simulink model "rigPeripheralNet"  (R2012b)
settings: Solver=FixedStepDiscrete  StartTime=0.0  StopTime=10.0  FixedStep=0.001  RelTol=1e-3
undefined symbols (not defined in the file): macaddr, modelConstants
libraries: xpcethernetlib x17, dspmtrx3 x6, simulink x5, xpcnetworkbufferlib x4, Lib_FileLogger x1
(part 1 of 2)
settings Model: xpc_rtwmakecfg_data=_xpcetherlib__xpcether8255xlib__xpcetherGbElib__xpcnblib_  BufferReuse=off  Creator=gilja  LastModifiedBy=NPTL
settings SolverCC: EnableConcurrentExecution=on  ConcurrentTasks=on
settings DataIOCC: SaveOutput=off  SignalLogging=off  SaveTime=off
settings OptimizationCC: InlineParams=on  InlineInvariantSignals=on  OptimizeBlockIOStorage=off  BufferReuse=off  ExpressionFolding=off  LocalBlockOutputs=off  SimCompilerOptimization=On
settings HardwareCC: ProdIntDivRoundTo=Zero  ProdEndianess=LittleEndian  ProdHWDeviceType=Generic->32-bit x86 compatible
settings ModelReferenceCC: ModelReferenceNumInstancesAllowed=Single  ModelReferenceMinAlgLoopOccurrences=on
settings RTWCC: SystemTargetFile=xpctarget.tlc  TemplateMakefile=xpc_default_tmf  Description=xPC Target  ProcessScript=xpctarget_make_rtw_hook  RTWCompilerOptimization=On
settings CodeAppCC: MaxIdLength=62
settings xpcTargetCC: TargetFcnLib=ansi_tfl_table_tmw.mat  CodeReplacementLibrary=XPC_BLAS  ParMdlRefBuildCompliant=on  ConcurrentExecutionCompliant=on  CombineSignalStateStructs=off  GRTInterface=on  xPCTaskExecutionProfile=on  xPCRL32EventNumber=5000  xPCisDownloadable=off  xPCLoadParamSetFile=off  xPCConcurrentTasks=off  xPCEnableSFAnimation=off

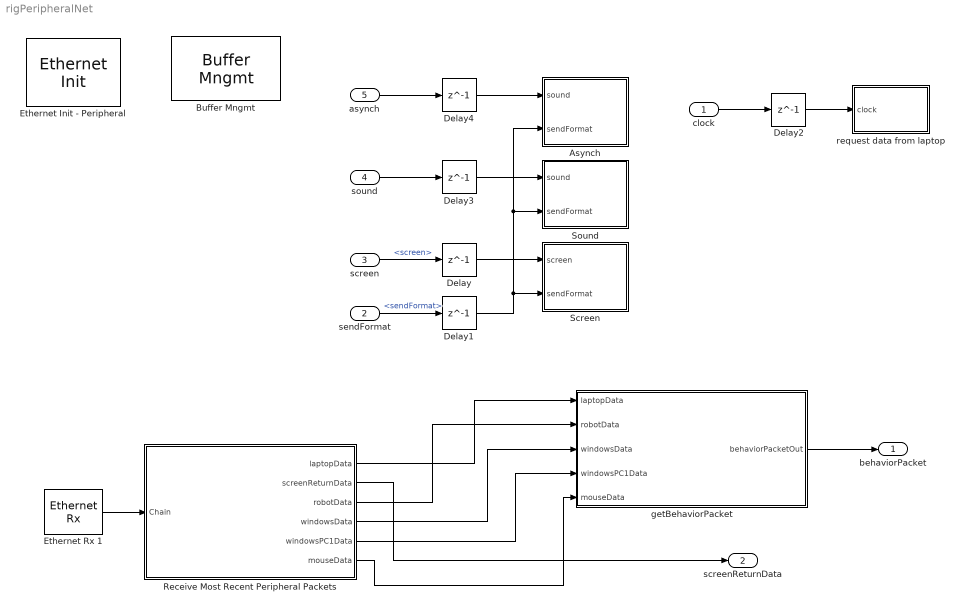
== system rigPeripheralNet ==
  clock : Inport  OutDataTypeStr=uint32
  sendFormat : Inport  Port=2  OutDataTypeStr=boolean
  screen : Inport  Port=3  OutDataTypeStr=Bus: fileLoggerFormatAndData  BusOutputAsStruct=on
  sound : Inport  Port=4  OutDataTypeStr=Bus: fileLoggerFormatAndData  BusOutputAsStruct=on
  asynch : Inport  Port=5  OutDataTypeStr=Bus: fileLoggerFormatAndData  BusOutputAsStruct=on
  Asynch : Subsystem
  "Buffer Mngmt " : xpcnetworkbufferlib/Buffer Mngmt   Priority=-1  SampleTime=-1  PoolSizes=modelConstants.networkBufferPoolSizes  ShowTune=on
  Delay{,1..4} (5 alike) : Delay  DelayLength=1  InitialCondition=0
  Ethernet Init - Peripheral : xpcethernetlib/Ethernet Init   Priority=-1  ID=3  Driver=Intel Gigabit  Bus=modelConstants.xpcNICConfig.peripheral.bus  Slot=modelConstants.xpcNICConfig.peripheral.slot  SampleTime=-1  AddressSource=Specify  MAC=macaddr('00:00:00:00:00:00')  TxSA=off  RxPromiscuous=off  Multicast={}  RxBad=off  RxShort=off  MaxMTU=1518  TxThreshold=10  TxBuffers=128  RxBuffers=8  ShowTune=on  NumRxBlks=1
  Ethernet Rx 1 : xpcethernetlib/Ethernet Rx   ID=3  SampleTime=modelConstants.sampleTime  Criteria=Receive all unmatched types [0 to 65535]  EtherType=[hex2dec('0000')]  BlkID=0
  Receive Most Recent Peripheral Packets : Subsystem
  Screen : Subsystem
  Sound : Subsystem
  getBehaviorPacket : MATLAB Function  TreatAsAtomicUnit=on
  request data from laptop : Subsystem
  behaviorPacket : Outport  OutDataTypeStr=Bus: behaviorPacketBus  BusOutputAsStruct=on
  screenReturnData : Outport  Port=2  OutDataTypeStr=Bus: peripheralData  BusOutputAsStruct=on
  wires:
  Ethernet Rx 1/1 -> Receive Most Recent Peripheral Packets/1(Chain)
  clock/1 -> Delay2/1
  Receive Most Recent Peripheral Packets/2(screenReturnData) -> screenReturnData/1
  sendFormat/1 -> Delay1/1  "<sendFormat>"
  screen/1 -> Delay/1  "<screen>"
  Delay/1 -> Screen/1(screen)
  Delay1/1 -> Asynch/2(sendFormat), Sound/2(sendFormat), Screen/2(sendFormat)
  Delay2/1 -> request data from laptop/1(clock)
  sound/1 -> Delay3/1
  Delay3/1 -> Sound/1(sound)
  asynch/1 -> Delay4/1
  Delay4/1 -> Asynch/1(sound)
  Receive Most Recent Peripheral Packets/1(laptopData) -> getBehaviorPacket/1(laptopData)
  Receive Most Recent Peripheral Packets/3(robotData) -> getBehaviorPacket/2(robotData)
  getBehaviorPacket/1(behaviorPacketOut) -> behaviorPacket/1
  Receive Most Recent Peripheral Packets/4(windowsData) -> getBehaviorPacket/3(windowsData)
  Receive Most Recent Peripheral Packets/5(windowsPC1Data) -> getBehaviorPacket/4(windowsPC1Data)
  Receive Most Recent Peripheral Packets/6(mouseData) -> getBehaviorPacket/5(mouseData)

== system rigPeripheralNet/Asynch ==
  sound : Inport  OutDataTypeStr=Bus: fileLoggerFormatAndData
  sendFormat : Inport  Port=2  OutDataTypeStr=boolean
  Asynch - Control : Subsystem
  Asynch - Data : Subsystem
  Bus Selector6 : BusSelector  OutputSignals=data.send,data.data,data.dataLen,format.format,format.formatLen
  Digital Clock : DigitalClock  SampleTime=0.001
  Logical Operator : Logic  AllPortsSameDT=off  OutDataTypeStr=boolean
  Logical Operator1 : Logic  AllPortsSameDT=off  OutDataTypeStr=boolean
  Wait 100 ms : simulink/Logic and Bit Operations/Compare To Constant  relop=>  const=0.4  OutDataTypeStr=boolean
  wires:
  Bus Selector6/3 -> Asynch - Data/2(dataLen)  "<dataLen>"
  Bus Selector6/2 -> Asynch - Data/1(data)  "<data>"
  Bus Selector6/1 -> Logical Operator1/2  "<send>"
  Bus Selector6/5 -> Asynch - Control/2(dataLen)  "<formatLen>"
  sound/1 -> Bus Selector6/1
  Bus Selector6/4 -> Asynch - Control/1(data)  "<format>"
  sendFormat/1 -> Logical Operator/2
  Wait 100 ms/1 -> Logical Operator/1, Logical Operator1/1
  Digital Clock/1 -> Wait 100 ms/1
  Logical Operator/1 -> Asynch - Control/Enable
  Logical Operator1/1 -> Asynch - Data/Enable

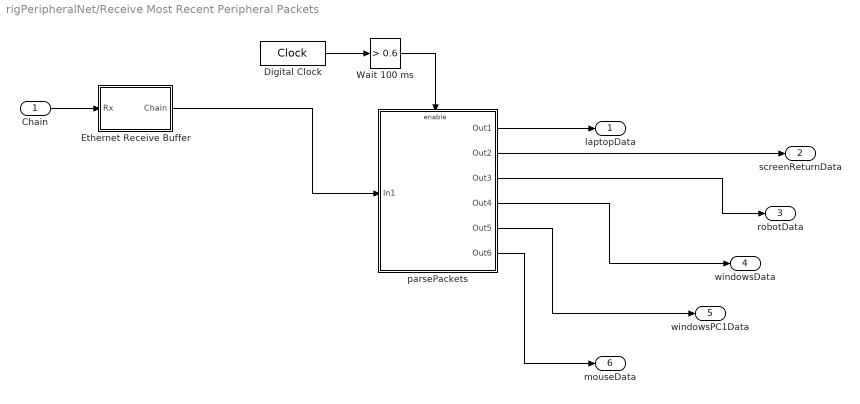
== system rigPeripheralNet/Receive Most Recent Peripheral Packets ==
  Chain : Inport
  Digital Clock : DigitalClock  SampleTime=0.001
  Ethernet Receive Buffer : Subsystem
  Wait 100 ms : simulink/Logic and Bit Operations/Compare To Constant  relop=>  const=0.6  OutDataTypeStr=boolean
  parsePackets : Subsystem
  laptopData : Outport  OutDataTypeStr=Bus: peripheralData
  screenReturnData : Outport  Port=2  OutDataTypeStr=Bus: peripheralData
  robotData : Outport  Port=3  OutDataTypeStr=Bus: peripheralData
  windowsData : Outport  Port=4  OutDataTypeStr=Bus: peripheralData
  windowsPC1Data : Outport  Port=5  OutDataTypeStr=Bus: peripheralData
  mouseData : Outport  Port=6  OutDataTypeStr=Bus: peripheralData
  wires:
  Chain/1 -> Ethernet Receive Buffer/1(Rx)
  Wait 100 ms/1 -> parsePackets/Enable
  Digital Clock/1 -> Wait 100 ms/1
  Ethernet Receive Buffer/1(Chain) -> parsePackets/1(In1)
  parsePackets/1(Out1) -> laptopData/1
  parsePackets/2(Out2) -> screenReturnData/1
  parsePackets/3(Out3) -> robotData/1
  parsePackets/4(Out4) -> windowsData/1
  parsePackets/5(Out5) -> windowsPC1Data/1
  parsePackets/6(Out6) -> mouseData/1

== system rigPeripheralNet/Screen ==
  screen : Inport  OutDataTypeStr=Bus: fileLoggerFormatAndData
  sendFormat : Inport  Port=2  OutDataTypeStr=boolean
  Bus Selector6 : BusSelector  OutputSignals=data.send,data.data,data.dataLen,format.format,format.formatLen
  Digital Clock : DigitalClock  SampleTime=0.001
  Logical Operator : Logic  AllPortsSameDT=off  OutDataTypeStr=boolean
  Logical Operator1 : Logic  AllPortsSameDT=off  OutDataTypeStr=boolean
  Screen - Control : Subsystem
  Screen - Data : Subsystem
  Wait 400 ms xPC has memory intialization issues early in the task : simulink/Logic and Bit Operations/Compare To Constant  relop=>  const=0.4  OutDataTypeStr=boolean
  wires:
  Bus Selector6/3 -> Screen - Data/2(dataLen)  "<dataLen>"
  Bus Selector6/2 -> Screen - Data/1(data)  "<data>"
  Bus Selector6/1 -> Logical Operator/2  "<send>"
  Bus Selector6/5 -> Screen - Control/2(dataLen)  "<formatLen>"
  screen/1 -> Bus Selector6/1
  Bus Selector6/4 -> Screen - Control/1(data)  "<format>"
  sendFormat/1 -> Logical Operator1/2
  Logical Operator/1 -> Screen - Data/Enable
  Logical Operator1/1 -> Screen - Control/Enable
  Digital Clock/1 -> Wait 400 ms xPC has memory intialization issues early in the task/1
  Wait 400 ms xPC has memory intialization issues early in the task/1 -> Logical Operator1/1, Logical Operator/1

== system rigPeripheralNet/Sound ==
  sound : Inport  OutDataTypeStr=Bus: fileLoggerFormatAndData
  sendFormat : Inport  Port=2  OutDataTypeStr=boolean
  Bus Selector6 : BusSelector  OutputSignals=data.send,data.data,data.dataLen,format.format,format.formatLen
  Digital Clock : DigitalClock  SampleTime=0.001
  Logical Operator : Logic  AllPortsSameDT=off  OutDataTypeStr=boolean
  Logical Operator1 : Logic  AllPortsSameDT=off  OutDataTypeStr=boolean
  Sound - Control : Subsystem
  Sound - Data : Subsystem
  Wait 100 ms : simulink/Logic and Bit Operations/Compare To Constant  relop=>  const=0.4  OutDataTypeStr=boolean
  wires:
  Bus Selector6/3 -> Sound - Data/2(dataLen)  "<dataLen>"
  Bus Selector6/2 -> Sound - Data/1(data)  "<data>"
  Bus Selector6/1 -> Logical Operator/2  "<send>"
  Bus Selector6/5 -> Sound - Control/2(dataLen)  "<formatLen>"
  sound/1 -> Bus Selector6/1
  Bus Selector6/4 -> Sound - Control/1(data)  "<format>"
  sendFormat/1 -> Logical Operator1/2
  Digital Clock/1 -> Wait 100 ms/1
  Wait 100 ms/1 -> Logical Operator1/1, Logical Operator/1
  Logical Operator/1 -> Sound - Data/Enable
  Logical Operator1/1 -> Sound - Control/Enable

== system rigPeripheralNet/request data from laptop ==
  clock : Inport
  Digital Clock : DigitalClock  SampleTime=0.001
  Laptop Data Request : MATLAB Function  TreatAsAtomicUnit=on
  Logical Operator : Logic  AllPortsSameDT=off  OutDataTypeStr=boolean
  UDP to Laptop : Subsystem
  Wait 100 ms : simulink/Logic and Bit Operations/Compare To Constant  relop=>  const=0.4  OutDataTypeStr=boolean
  wires:
  Laptop Data Request/3(dataLen) -> UDP to Laptop/2(udpDataLen)
  Laptop Data Request/2(data) -> UDP to Laptop/1(udpData)
  Logical Operator/1 -> UDP to Laptop/Enable
  clock/1 -> Laptop Data Request/1(clock)
  Digital Clock/1 -> Wait 100 ms/1
  Wait 100 ms/1 -> Logical Operator/1
  Laptop Data Request/1(send) -> Logical Operator/2

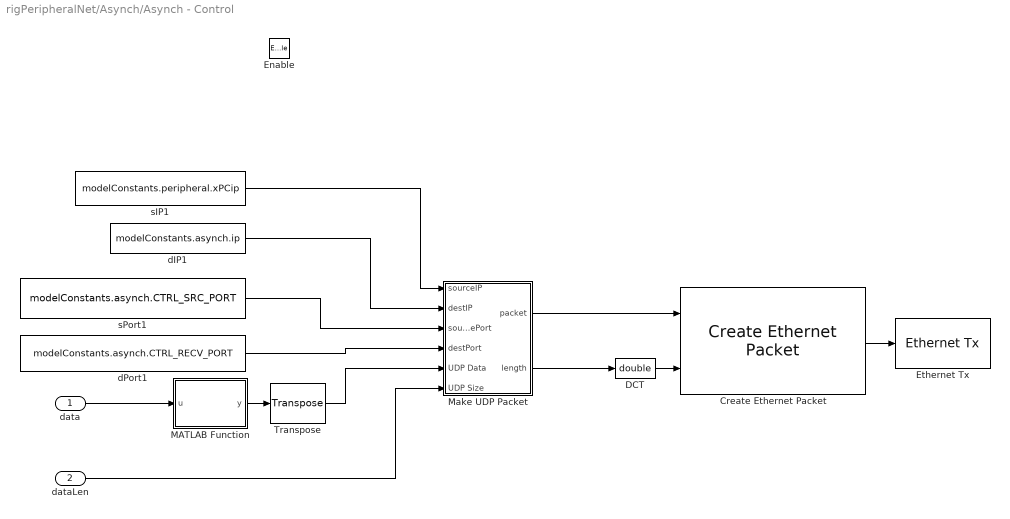
== system rigPeripheralNet/Asynch/Asynch - Control ==
  data : Inport
  dataLen : Inport  Port=2
  Enable : EnablePort
  "Create Ethernet Packet " : xpcethernetlib/Create Ethernet Packet   DstMac=macaddr('FF:FF:FF:FF:FF:FF')  EtherType=hex2dec('0800')
  DCT : DataTypeConversion  OutDataTypeStr=double
  "Ethernet Tx " : xpcethernetlib/Ethernet Tx   ID=3  SampleTime=-1
  MATLAB Function : MATLAB Function  TreatAsAtomicUnit=on
  Make UDP Packet : Subsystem
  Transpose : dspmtrx3/Transpose  Hermitian=off  overflowFlag=off
  dIP1 : Constant  Value=modelConstants.asynch.ip  OutDataTypeStr=uint8
  dPort1 : Constant  Value=modelConstants.asynch.CTRL_RECV_PORT  OutDataTypeStr=uint16
  sIP1 : Constant  Value=modelConstants.peripheral.xPCip  OutDataTypeStr=uint8
  sPort1 : Constant  Value=modelConstants.asynch.CTRL_SRC_PORT  OutDataTypeStr=uint16
  wires:
  dPort1/1 -> Make UDP Packet/4(destPort)
  Make UDP Packet/2(length) -> DCT/1
  "Create Ethernet Packet "/1 -> "Ethernet Tx "/1
  Make UDP Packet/1(packet) -> "Create Ethernet Packet "/1
  DCT/1 -> "Create Ethernet Packet "/2
  data/1 -> MATLAB Function/1(u)
  MATLAB Function/1(y) -> Transpose/1
  dataLen/1 -> Make UDP Packet/6(UDP Size)
  sPort1/1 -> Make UDP Packet/3(sourcePort)
  dIP1/1 -> Make UDP Packet/2(destIP)
  sIP1/1 -> Make UDP Packet/1(sourceIP)
  Transpose/1 -> Make UDP Packet/5(UDP Data)

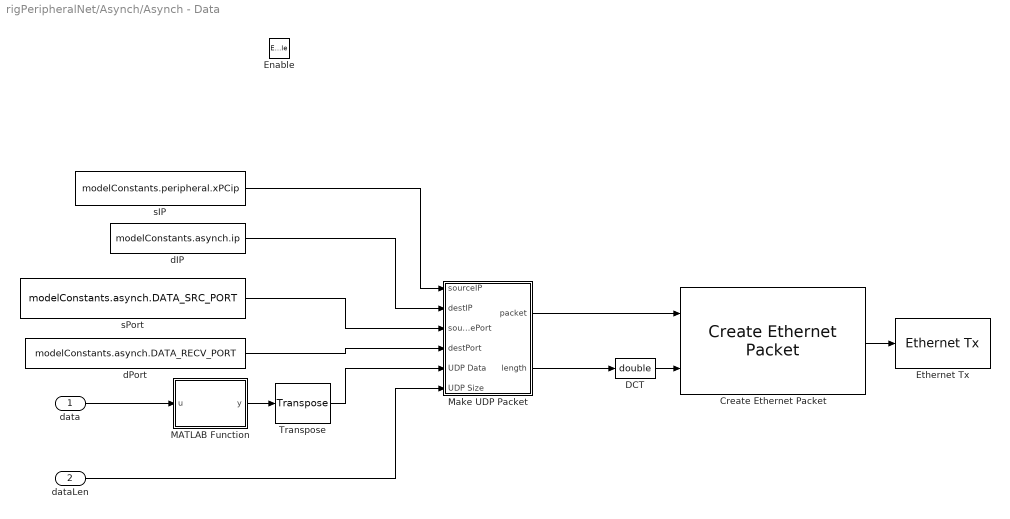
== system rigPeripheralNet/Asynch/Asynch - Data ==
  data : Inport
  dataLen : Inport  Port=2
  Enable : EnablePort
  "Create Ethernet Packet " : xpcethernetlib/Create Ethernet Packet   DstMac=macaddr('FF:FF:FF:FF:FF:FF')  EtherType=hex2dec('0800')
  DCT : DataTypeConversion  OutDataTypeStr=double
  "Ethernet Tx " : xpcethernetlib/Ethernet Tx   ID=3  SampleTime=-1
  MATLAB Function : MATLAB Function  TreatAsAtomicUnit=on
  Make UDP Packet : Subsystem
  Transpose : dspmtrx3/Transpose  Hermitian=off  overflowFlag=off
  dIP : Constant  Value=modelConstants.asynch.ip  OutDataTypeStr=uint8
  dPort : Constant  Value=modelConstants.asynch.DATA_RECV_PORT  OutDataTypeStr=uint16
  sIP : Constant  Value=modelConstants.peripheral.xPCip  OutDataTypeStr=uint8
  sPort : Constant  Value=modelConstants.asynch.DATA_SRC_PORT  OutDataTypeStr=uint16
  wires:
  dPort/1 -> Make UDP Packet/4(destPort)
  Make UDP Packet/2(length) -> DCT/1
  "Create Ethernet Packet "/1 -> "Ethernet Tx "/1
  Make UDP Packet/1(packet) -> "Create Ethernet Packet "/1
  DCT/1 -> "Create Ethernet Packet "/2
  data/1 -> MATLAB Function/1(u)
  MATLAB Function/1(y) -> Transpose/1
  dataLen/1 -> Make UDP Packet/6(UDP Size)
  sPort/1 -> Make UDP Packet/3(sourcePort)
  dIP/1 -> Make UDP Packet/2(destIP)
  sIP/1 -> Make UDP Packet/1(sourceIP)
  Transpose/1 -> Make UDP Packet/5(UDP Data)

== system rigPeripheralNet/Receive Most Recent Peripheral Packets/Ethernet Receive Buffer ==
  note: HACK: HARDCODED CHAIN BUFFER AT 39
      | Affects NB Buffering Block & NB Unlink
  Rx : Inport
  Buffer : xpcnetworkbufferlib/Buffer   ChainSize=38  BufferSize=0  Threshold=0
  Bus Creator : BusCreator  Inputs=2
  "Chain Size " : xpcnetworkbufferlib/Chain Size 
  Chain : Outport
  wires:
  Buffer/1 -> Bus Creator/1  "Buffers"
  Bus Creator/1 -> Chain/1
  "Chain Size "/2 -> Bus Creator/2  "Chain Size"
  Rx/1 -> "Chain Size "/1
  "Chain Size "/1 -> Buffer/1

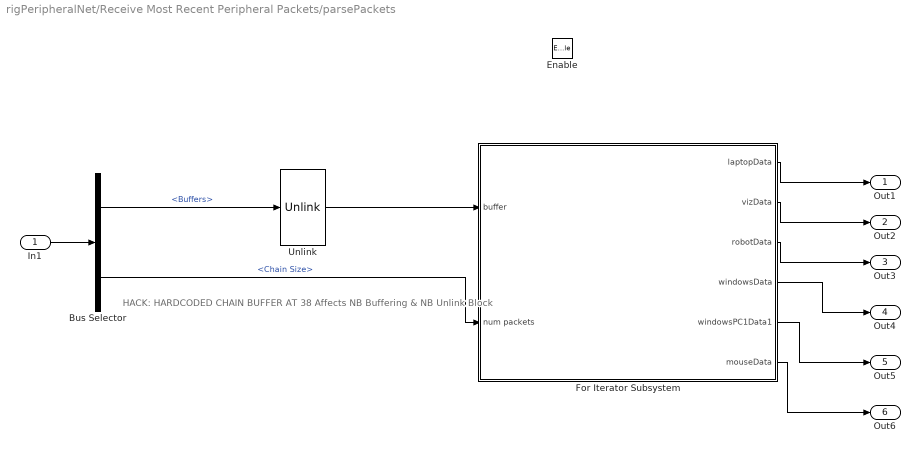
== system rigPeripheralNet/Receive Most Recent Peripheral Packets/parsePackets ==
  note: HACK: HARDCODED CHAIN BUFFER AT 38
      | Affects NB Buffering & NB Unlink Block
  In1 : Inport
  Enable : EnablePort
  Bus Selector : BusSelector  OutputSignals=Buffers,Chain Size
  For Iterator Subsystem : Subsystem  TreatAsAtomicUnit=on
  "Unlink " : xpcnetworkbufferlib/Unlink   VectorLength=38
  Out1 : Outport
  Out2 : Outport  Port=2
  Out3 : Outport  Port=3
  Out4 : Outport  Port=4
  Out5 : Outport  Port=5  OutDataTypeStr=Bus: peripheralData
  Out6 : Outport  Port=6  OutDataTypeStr=Bus: peripheralData
  wires:
  In1/1 -> Bus Selector/1
  For Iterator Subsystem/1(laptopData) -> Out1/1
  For Iterator Subsystem/2(vizData) -> Out2/1
  "Unlink "/1 -> For Iterator Subsystem/1(buffer)
  Bus Selector/1 -> "Unlink "/1  "<Buffers>"
  For Iterator Subsystem/3(robotData) -> Out3/1
  Bus Selector/2 -> For Iterator Subsystem/2(num packets)  "<Chain Size>"
  For Iterator Subsystem/4(windowsData) -> Out4/1
  For Iterator Subsystem/5(windowsPC1Data1) -> Out5/1
  For Iterator Subsystem/6(mouseData) -> Out6/1

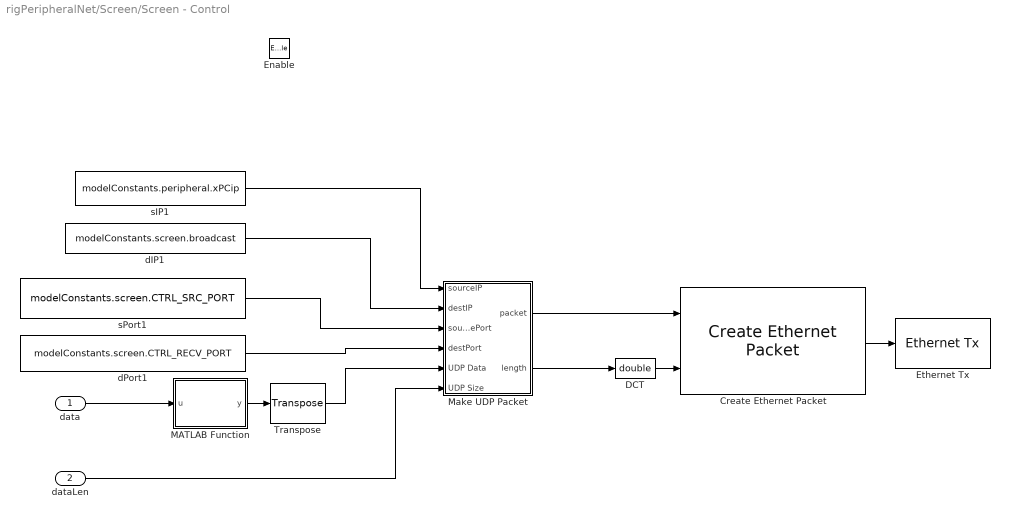
== system rigPeripheralNet/Screen/Screen - Control ==
  data : Inport
  dataLen : Inport  Port=2
  Enable : EnablePort
  "Create Ethernet Packet " : xpcethernetlib/Create Ethernet Packet   DstMac=macaddr('FF:FF:FF:FF:FF:FF')  EtherType=hex2dec('0800')
  DCT : DataTypeConversion  OutDataTypeStr=double
  "Ethernet Tx " : xpcethernetlib/Ethernet Tx   ID=3  SampleTime=-1
  MATLAB Function : MATLAB Function  TreatAsAtomicUnit=on
  Make UDP Packet : Subsystem
  Transpose : dspmtrx3/Transpose  Hermitian=off  overflowFlag=off
  dIP1 : Constant  Value=modelConstants.screen.broadcast  OutDataTypeStr=uint8
  dPort1 : Constant  Value=modelConstants.screen.CTRL_RECV_PORT  OutDataTypeStr=uint16
  sIP1 : Constant  Value=modelConstants.peripheral.xPCip  OutDataTypeStr=uint8
  sPort1 : Constant  Value=modelConstants.screen.CTRL_SRC_PORT  OutDataTypeStr=uint16
  wires:
  dPort1/1 -> Make UDP Packet/4(destPort)
  Make UDP Packet/2(length) -> DCT/1
  "Create Ethernet Packet "/1 -> "Ethernet Tx "/1
  Make UDP Packet/1(packet) -> "Create Ethernet Packet "/1
  DCT/1 -> "Create Ethernet Packet "/2
  data/1 -> MATLAB Function/1(u)
  MATLAB Function/1(y) -> Transpose/1
  dataLen/1 -> Make UDP Packet/6(UDP Size)
  sPort1/1 -> Make UDP Packet/3(sourcePort)
  dIP1/1 -> Make UDP Packet/2(destIP)
  sIP1/1 -> Make UDP Packet/1(sourceIP)
  Transpose/1 -> Make UDP Packet/5(UDP Data)

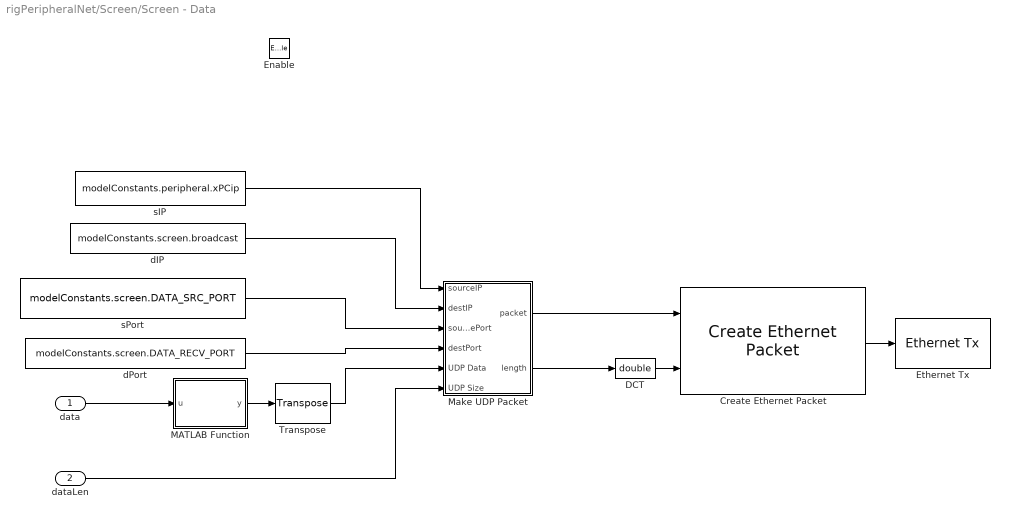
== system rigPeripheralNet/Screen/Screen - Data ==
  data : Inport
  dataLen : Inport  Port=2
  Enable : EnablePort
  "Create Ethernet Packet " : xpcethernetlib/Create Ethernet Packet   DstMac=macaddr('FF:FF:FF:FF:FF:FF')  EtherType=hex2dec('0800')
  DCT : DataTypeConversion  OutDataTypeStr=double
  "Ethernet Tx " : xpcethernetlib/Ethernet Tx   ID=3  SampleTime=-1
  MATLAB Function : MATLAB Function  TreatAsAtomicUnit=on
  Make UDP Packet : Subsystem
  Transpose : dspmtrx3/Transpose  Hermitian=off  overflowFlag=off
  dIP : Constant  Value=modelConstants.screen.broadcast  OutDataTypeStr=uint8
  dPort : Constant  Value=modelConstants.screen.DATA_RECV_PORT  OutDataTypeStr=uint16
  sIP : Constant  Value=modelConstants.peripheral.xPCip  OutDataTypeStr=uint8
  sPort : Constant  Value=modelConstants.screen.DATA_SRC_PORT  OutDataTypeStr=uint16
  wires:
  dPort/1 -> Make UDP Packet/4(destPort)
  Make UDP Packet/2(length) -> DCT/1
  "Create Ethernet Packet "/1 -> "Ethernet Tx "/1
  Make UDP Packet/1(packet) -> "Create Ethernet Packet "/1
  DCT/1 -> "Create Ethernet Packet "/2
  data/1 -> MATLAB Function/1(u)
  MATLAB Function/1(y) -> Transpose/1
  dataLen/1 -> Make UDP Packet/6(UDP Size)
  sPort/1 -> Make UDP Packet/3(sourcePort)
  dIP/1 -> Make UDP Packet/2(destIP)
  sIP/1 -> Make UDP Packet/1(sourceIP)
  Transpose/1 -> Make UDP Packet/5(UDP Data)

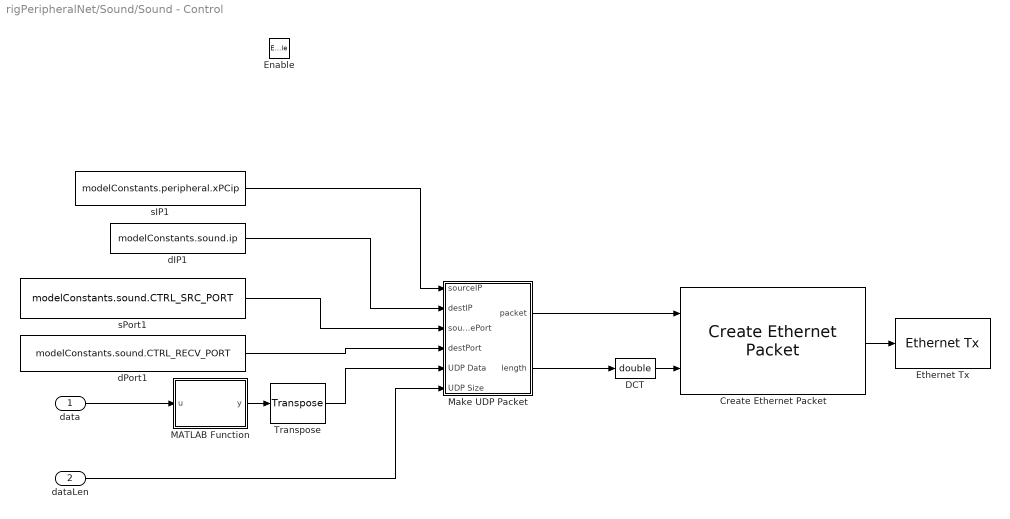
== system rigPeripheralNet/Sound/Sound - Control ==
  data : Inport
  dataLen : Inport  Port=2
  Enable : EnablePort
  "Create Ethernet Packet " : xpcethernetlib/Create Ethernet Packet   DstMac=macaddr('FF:FF:FF:FF:FF:FF')  EtherType=hex2dec('0800')
  DCT : DataTypeConversion  OutDataTypeStr=double
  "Ethernet Tx " : xpcethernetlib/Ethernet Tx   ID=3  SampleTime=-1
  MATLAB Function : MATLAB Function  TreatAsAtomicUnit=on
  Make UDP Packet : Subsystem
  Transpose : dspmtrx3/Transpose  Hermitian=off  overflowFlag=off
  dIP1 : Constant  Value=modelConstants.sound.ip  OutDataTypeStr=uint8
  dPort1 : Constant  Value=modelConstants.sound.CTRL_RECV_PORT  OutDataTypeStr=uint16
  sIP1 : Constant  Value=modelConstants.peripheral.xPCip  OutDataTypeStr=uint8
  sPort1 : Constant  Value=modelConstants.sound.CTRL_SRC_PORT  OutDataTypeStr=uint16
  wires:
  dPort1/1 -> Make UDP Packet/4(destPort)
  Make UDP Packet/2(length) -> DCT/1
  "Create Ethernet Packet "/1 -> "Ethernet Tx "/1
  Make UDP Packet/1(packet) -> "Create Ethernet Packet "/1
  DCT/1 -> "Create Ethernet Packet "/2
  data/1 -> MATLAB Function/1(u)
  MATLAB Function/1(y) -> Transpose/1
  dataLen/1 -> Make UDP Packet/6(UDP Size)
  sPort1/1 -> Make UDP Packet/3(sourcePort)
  dIP1/1 -> Make UDP Packet/2(destIP)
  sIP1/1 -> Make UDP Packet/1(sourceIP)
  Transpose/1 -> Make UDP Packet/5(UDP Data)

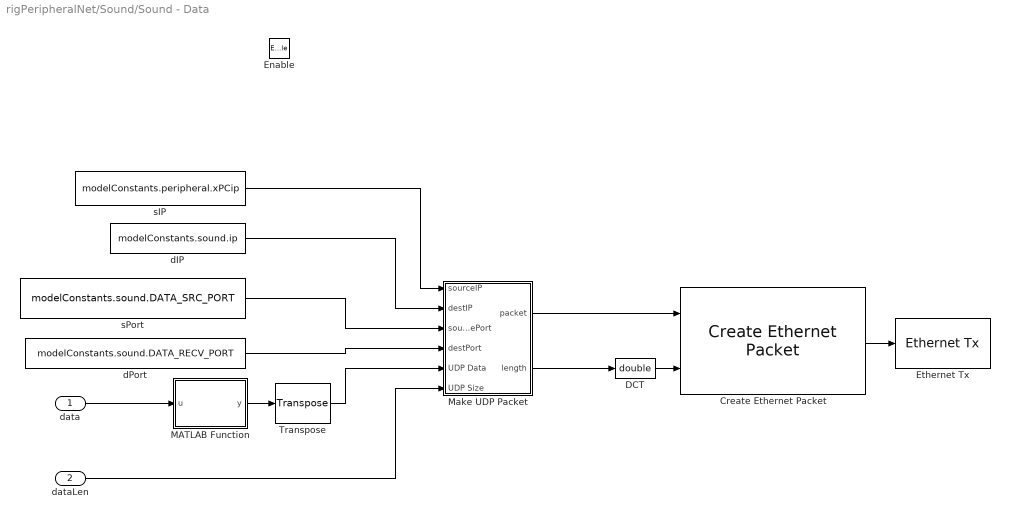
== system rigPeripheralNet/Sound/Sound - Data ==
  data : Inport
  dataLen : Inport  Port=2
  Enable : EnablePort
  "Create Ethernet Packet " : xpcethernetlib/Create Ethernet Packet   DstMac=macaddr('FF:FF:FF:FF:FF:FF')  EtherType=hex2dec('0800')
  DCT : DataTypeConversion  OutDataTypeStr=double
  "Ethernet Tx " : xpcethernetlib/Ethernet Tx   ID=3  SampleTime=-1
  MATLAB Function : MATLAB Function  TreatAsAtomicUnit=on
  Make UDP Packet : Subsystem
  Transpose : dspmtrx3/Transpose  Hermitian=off  overflowFlag=off
  dIP : Constant  Value=modelConstants.sound.ip  OutDataTypeStr=uint8
  dPort : Constant  Value=modelConstants.sound.DATA_RECV_PORT  OutDataTypeStr=uint16
  sIP : Constant  Value=modelConstants.peripheral.xPCip  OutDataTypeStr=uint8
  sPort : Constant  Value=modelConstants.sound.DATA_SRC_PORT  OutDataTypeStr=uint16
  wires:
  dPort/1 -> Make UDP Packet/4(destPort)
  Make UDP Packet/2(length) -> DCT/1
  "Create Ethernet Packet "/1 -> "Ethernet Tx "/1
  Make UDP Packet/1(packet) -> "Create Ethernet Packet "/1
  DCT/1 -> "Create Ethernet Packet "/2
  data/1 -> MATLAB Function/1(u)
  MATLAB Function/1(y) -> Transpose/1
  dataLen/1 -> Make UDP Packet/6(UDP Size)
  sPort/1 -> Make UDP Packet/3(sourcePort)
  dIP/1 -> Make UDP Packet/2(destIP)
  sIP/1 -> Make UDP Packet/1(sourceIP)
  Transpose/1 -> Make UDP Packet/5(UDP Data)

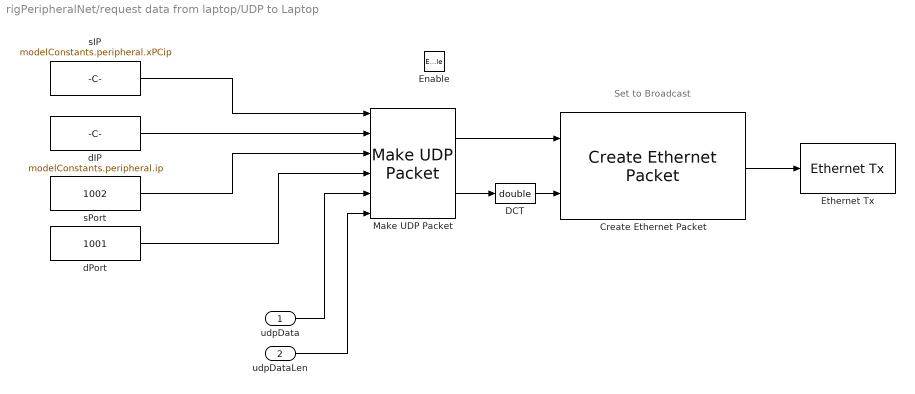
== system rigPeripheralNet/request data from laptop/UDP to Laptop ==
  note: Set to Broadcast
  udpData : Inport
  udpDataLen : Inport  Port=2
  Enable : EnablePort
  "Create Ethernet Packet " : xpcethernetlib/Create Ethernet Packet   DstMac=macaddr('FF:FF:FF:FF:FF:FF')  EtherType=hex2dec('0800')
  DCT : DataTypeConversion  OutDataTypeStr=double
  "Ethernet Tx " : xpcethernetlib/Ethernet Tx   ID=3  SampleTime=-1
  Make UDP Packet : Lib_FileLogger/Fille Logger/Make UDP Packet
  dIP : Constant  Value=modelConstants.peripheral.ip  OutDataTypeStr=uint8
  dPort : Constant  Value=1001  OutDataTypeStr=uint16
  sIP : Constant  Value=modelConstants.peripheral.xPCip  OutDataTypeStr=uint8
  sPort : Constant  Value=1002  OutDataTypeStr=uint16
  wires:
  dPort/1 -> Make UDP Packet/4
  sIP/1 -> Make UDP Packet/1
  Make UDP Packet/2 -> DCT/1
  Make UDP Packet/1 -> "Create Ethernet Packet "/1
  DCT/1 -> "Create Ethernet Packet "/2
  dIP/1 -> Make UDP Packet/2
  sPort/1 -> Make UDP Packet/3
  udpDataLen/1 -> Make UDP Packet/6
  "Create Ethernet Packet "/1 -> "Ethernet Tx "/1
  udpData/1 -> Make UDP Packet/5

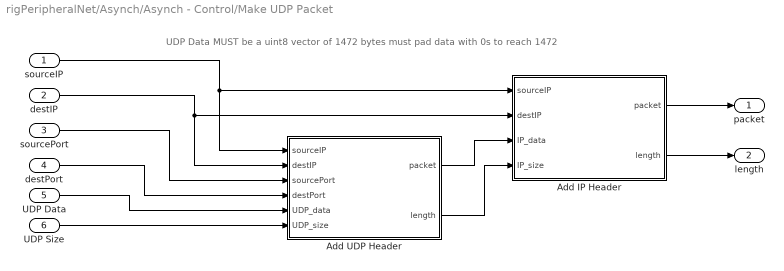
== system rigPeripheralNet/Asynch/Asynch - Control/Make UDP Packet ==
  note: UDP Data MUST be a uint8 vector of 1472 bytes
      | must pad data with 0s to reach 1472
  sourceIP : Inport
  destIP : Inport  Port=2
  sourcePort : Inport  Port=3
  destPort : Inport  Port=4
  UDP Data : Inport  Port=5
  UDP Size : Inport  Port=6
  Add IP Header : MATLAB Function  TreatAsAtomicUnit=on
  Add UDP Header : MATLAB Function  TreatAsAtomicUnit=on
  packet : Outport
  length : Outport  Port=2
  wires:
  Add UDP Header/2(length) -> Add IP Header/4(IP_size)
  Add UDP Header/1(packet) -> Add IP Header/3(IP_data)
  sourceIP/1 -> Add UDP Header/1(sourceIP), Add IP Header/1(sourceIP)
  destIP/1 -> Add UDP Header/2(destIP), Add IP Header/2(destIP)
  sourcePort/1 -> Add UDP Header/3(sourcePort)
  destPort/1 -> Add UDP Header/4(destPort)
  UDP Data/1 -> Add UDP Header/5(UDP_data)
  Add IP Header/1(packet) -> packet/1
  Add IP Header/2(length) -> length/1
  UDP Size/1 -> Add UDP Header/6(UDP_size)

== system rigPeripheralNet/Asynch/Asynch - Data/Make UDP Packet ==
  note: UDP Data MUST be a uint8 vector of 1472 bytes
      | must pad data with 0s to reach 1472
  sourceIP : Inport
  destIP : Inport  Port=2
  sourcePort : Inport  Port=3
  destPort : Inport  Port=4
  UDP Data : Inport  Port=5
  UDP Size : Inport  Port=6
  Add IP Header : MATLAB Function  TreatAsAtomicUnit=on
  Add UDP Header : MATLAB Function  TreatAsAtomicUnit=on
  packet : Outport
  length : Outport  Port=2
  wires:
  Add UDP Header/2(length) -> Add IP Header/4(IP_size)
  Add UDP Header/1(packet) -> Add IP Header/3(IP_data)
  sourceIP/1 -> Add UDP Header/1(sourceIP), Add IP Header/1(sourceIP)
  destIP/1 -> Add UDP Header/2(destIP), Add IP Header/2(destIP)
  sourcePort/1 -> Add UDP Header/3(sourcePort)
  destPort/1 -> Add UDP Header/4(destPort)
  UDP Data/1 -> Add UDP Header/5(UDP_data)
  Add IP Header/1(packet) -> packet/1
  Add IP Header/2(length) -> length/1
  UDP Size/1 -> Add UDP Header/6(UDP_size)

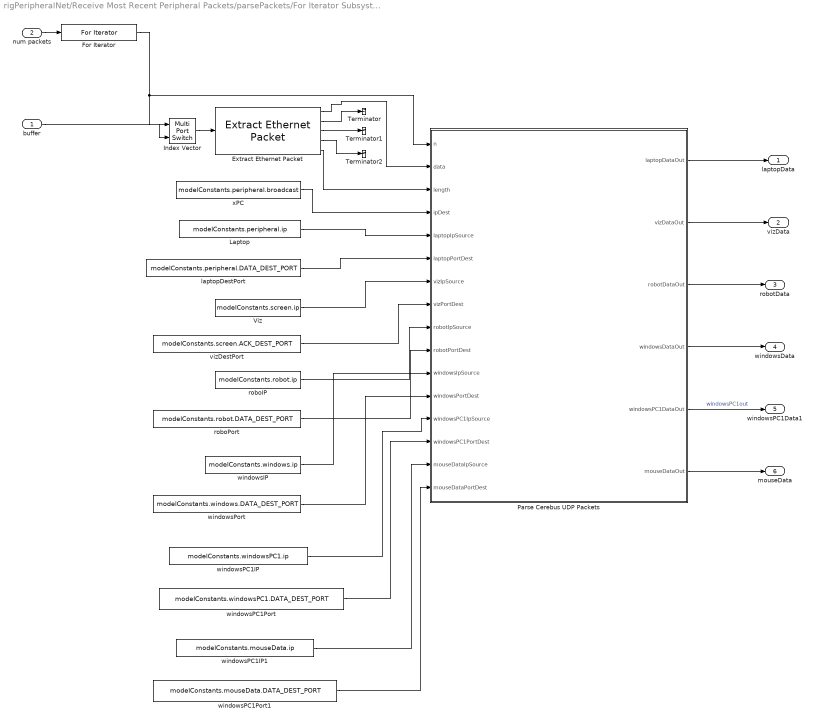
== system rigPeripheralNet/Receive Most Recent Peripheral Packets/parsePackets/For Iterator Subsystem ==
  buffer : Inport
  num packets : Inport  Port=2
  Extract Ethernet Packet : xpcethernetlib/Extract Ethernet Packet   EthernetDataSize=1400
  For Iterator : ForIterator  IterationSource=external  IterationVariableDataType=int8
  Index Vector : MultiPortSwitch  Inputs=1
  Laptop : Constant  Value=modelConstants.peripheral.ip  OutDataTypeStr=uint8
  Parse Cerebus UDP Packets : MATLAB Function  TreatAsAtomicUnit=on
  Terminator : Terminator
  Terminator1 : Terminator
  Terminator2 : Terminator
  Viz : Constant  Value=modelConstants.screen.ip  OutDataTypeStr=uint8
  laptopDestPort : Constant  Value=modelConstants.peripheral.DATA_DEST_PORT  OutDataTypeStr=uint16
  roboIP : Constant  Value=modelConstants.robot.ip  OutDataTypeStr=uint8
  roboPort : Constant  Value=modelConstants.robot.DATA_DEST_PORT  OutDataTypeStr=uint16
  vizDestPort : Constant  Value=modelConstants.screen.ACK_DEST_PORT  OutDataTypeStr=uint16
  windowsIP : Constant  Value=modelConstants.windows.ip  OutDataTypeStr=uint8
  windowsPC1IP : Constant  Value=modelConstants.windowsPC1.ip  OutDataTypeStr=uint8
  windowsPC1IP1 : Constant  Value=modelConstants.mouseData.ip  OutDataTypeStr=uint8
  windowsPC1Port : Constant  Value=modelConstants.windowsPC1.DATA_DEST_PORT  OutDataTypeStr=uint16
  windowsPC1Port1 : Constant  Value=modelConstants.mouseData.DATA_DEST_PORT  OutDataTypeStr=uint16
  windowsPort : Constant  Value=modelConstants.windows.DATA_DEST_PORT  OutDataTypeStr=uint16
  xPC : Constant  Value=modelConstants.peripheral.broadcast  OutDataTypeStr=uint8
  laptopData : Outport  OutDataTypeStr=Bus: peripheralData
  vizData : Outport  Port=2  OutDataTypeStr=Bus: peripheralData
  robotData : Outport  Port=3  OutDataTypeStr=Bus: peripheralData
  windowsData : Outport  Port=4  OutDataTypeStr=Bus: peripheralData
  windowsPC1Data1 : Outport  Port=5  OutDataTypeStr=Bus: peripheralData
  mouseData : Outport  Port=6  OutDataTypeStr=Bus: peripheralData
  wires:
  For Iterator/1 -> Parse Cerebus UDP Packets/1(n), Index Vector/1
  Extract Ethernet Packet/5 -> Parse Cerebus UDP Packets/3(length)
  num packets/1 -> For Iterator/1
  buffer/1 -> Index Vector/2
  Index Vector/1 -> Extract Ethernet Packet/1
  Extract Ethernet Packet/1 -> Parse Cerebus UDP Packets/2(data)
  Extract Ethernet Packet/2 -> Terminator/1
  Extract Ethernet Packet/3 -> Terminator1/1
  Extract Ethernet Packet/4 -> Terminator2/1
  Laptop/1 -> Parse Cerebus UDP Packets/5(laptopIpSource)
  xPC/1 -> Parse Cerebus UDP Packets/4(ipDest)
  laptopDestPort/1 -> Parse Cerebus UDP Packets/6(laptopPortDest)
  Parse Cerebus UDP Packets/1(laptopDataOut) -> laptopData/1
  Parse Cerebus UDP Packets/2(vizDataOut) -> vizData/1
  Viz/1 -> Parse Cerebus UDP Packets/7(vizIpSource)
  vizDestPort/1 -> Parse Cerebus UDP Packets/8(vizPortDest)
  roboIP/1 -> Parse Cerebus UDP Packets/9(robotIpSource)
  roboPort/1 -> Parse Cerebus UDP Packets/10(robotPortDest)
  Parse Cerebus UDP Packets/3(robotDataOut) -> robotData/1
  windowsIP/1 -> Parse Cerebus UDP Packets/11(windowsIpSource)
  windowsPort/1 -> Parse Cerebus UDP Packets/12(windowsPortDest)
  Parse Cerebus UDP Packets/4(windowsDataOut) -> windowsData/1
  windowsPC1IP/1 -> Parse Cerebus UDP Packets/13(windowsPC1IpSource)
  windowsPC1Port/1 -> Parse Cerebus UDP Packets/14(windowsPC1PortDest)
  Parse Cerebus UDP Packets/5(windowsPC1DataOut) -> windowsPC1Data1/1  "windowsPC1out"
  Parse Cerebus UDP Packets/6(mouseDataOut) -> mouseData/1
  windowsPC1IP1/1 -> Parse Cerebus UDP Packets/15(mouseDataIpSource)
  windowsPC1Port1/1 -> Parse Cerebus UDP Packets/16(mouseDataPortDest)

== system rigPeripheralNet/Screen/Screen - Control/Make UDP Packet ==
  note: UDP Data MUST be a uint8 vector of 1472 bytes
      | must pad data with 0s to reach 1472
  sourceIP : Inport
  destIP : Inport  Port=2
  sourcePort : Inport  Port=3
  destPort : Inport  Port=4
  UDP Data : Inport  Port=5
  UDP Size : Inport  Port=6
  Add IP Header : MATLAB Function  TreatAsAtomicUnit=on
  Add UDP Header : MATLAB Function  TreatAsAtomicUnit=on
  packet : Outport
  length : Outport  Port=2
  wires:
  Add UDP Header/2(length) -> Add IP Header/4(IP_size)
  Add UDP Header/1(packet) -> Add IP Header/3(IP_data)
  sourceIP/1 -> Add UDP Header/1(sourceIP), Add IP Header/1(sourceIP)
  destIP/1 -> Add UDP Header/2(destIP), Add IP Header/2(destIP)
  sourcePort/1 -> Add UDP Header/3(sourcePort)
  destPort/1 -> Add UDP Header/4(destPort)
  UDP Data/1 -> Add UDP Header/5(UDP_data)
  Add IP Header/1(packet) -> packet/1
  Add IP Header/2(length) -> length/1
  UDP Size/1 -> Add UDP Header/6(UDP_size)

== system rigPeripheralNet/Screen/Screen - Data/Make UDP Packet ==
  note: UDP Data MUST be a uint8 vector of 1472 bytes
      | must pad data with 0s to reach 1472
  sourceIP : Inport
  destIP : Inport  Port=2
  sourcePort : Inport  Port=3
  destPort : Inport  Port=4
  UDP Data : Inport  Port=5
  UDP Size : Inport  Port=6
  Add IP Header : MATLAB Function  TreatAsAtomicUnit=on
  Add UDP Header : MATLAB Function  TreatAsAtomicUnit=on
  packet : Outport
  length : Outport  Port=2
  wires:
  Add UDP Header/2(length) -> Add IP Header/4(IP_size)
  Add UDP Header/1(packet) -> Add IP Header/3(IP_data)
  sourceIP/1 -> Add UDP Header/1(sourceIP), Add IP Header/1(sourceIP)
  destIP/1 -> Add UDP Header/2(destIP), Add IP Header/2(destIP)
  sourcePort/1 -> Add UDP Header/3(sourcePort)
  destPort/1 -> Add UDP Header/4(destPort)
  UDP Data/1 -> Add UDP Header/5(UDP_data)
  Add IP Header/1(packet) -> packet/1
  Add IP Header/2(length) -> length/1
  UDP Size/1 -> Add UDP Header/6(UDP_size)

== system rigPeripheralNet/Sound/Sound - Control/Make UDP Packet ==
  note: UDP Data MUST be a uint8 vector of 1472 bytes
      | must pad data with 0s to reach 1472
  sourceIP : Inport
  destIP : Inport  Port=2
  sourcePort : Inport  Port=3
  destPort : Inport  Port=4
  UDP Data : Inport  Port=5
  UDP Size : Inport  Port=6
  Add IP Header : MATLAB Function  TreatAsAtomicUnit=on
  Add UDP Header : MATLAB Function  TreatAsAtomicUnit=on
  packet : Outport
  length : Outport  Port=2
  wires:
  Add UDP Header/2(length) -> Add IP Header/4(IP_size)
  Add UDP Header/1(packet) -> Add IP Header/3(IP_data)
  sourceIP/1 -> Add UDP Header/1(sourceIP), Add IP Header/1(sourceIP)
  destIP/1 -> Add UDP Header/2(destIP), Add IP Header/2(destIP)
  sourcePort/1 -> Add UDP Header/3(sourcePort)
  destPort/1 -> Add UDP Header/4(destPort)
  UDP Data/1 -> Add UDP Header/5(UDP_data)
  Add IP Header/1(packet) -> packet/1
  Add IP Header/2(length) -> length/1
  UDP Size/1 -> Add UDP Header/6(UDP_size)

== system rigPeripheralNet/Sound/Sound - Data/Make UDP Packet ==
  note: UDP Data MUST be a uint8 vector of 1472 bytes
      | must pad data with 0s to reach 1472
  sourceIP : Inport
  destIP : Inport  Port=2
  sourcePort : Inport  Port=3
  destPort : Inport  Port=4
  UDP Data : Inport  Port=5
  UDP Size : Inport  Port=6
  Add IP Header : MATLAB Function  TreatAsAtomicUnit=on
  Add UDP Header : MATLAB Function  TreatAsAtomicUnit=on
  packet : Outport
  length : Outport  Port=2
  wires:
  Add UDP Header/2(length) -> Add IP Header/4(IP_size)
  Add UDP Header/1(packet) -> Add IP Header/3(IP_data)
  sourceIP/1 -> Add UDP Header/1(sourceIP), Add IP Header/1(sourceIP)
  destIP/1 -> Add UDP Header/2(destIP), Add IP Header/2(destIP)
  sourcePort/1 -> Add UDP Header/3(sourcePort)
  destPort/1 -> Add UDP Header/4(destPort)
  UDP Data/1 -> Add UDP Header/5(UDP_data)
  Add IP Header/1(packet) -> packet/1
  Add IP Header/2(length) -> length/1
  UDP Size/1 -> Add UDP Header/6(UDP_size)

== matlab function rigPeripheralNet/Screen/Screen - Control/MATLAB Function ==
  data: u input; y output
function y = padData(u)

z = uint8(zeros(1434, 1))';

z(1:length(u)) = u;

y = z';

== matlab function rigPeripheralNet/Screen/Screen - Control/Make UDP Packet/Add IP Header ==
  data: sourceIP input uint8 size=[1 4]; packet output uint8; destIP input uint8 size=[1 4]; IP_data input uint8; IP_size input uint16 size=[1 1]; length output uint16 size=[1 1]
function [packet, length] = makeIP(sourceIP, destIP, IP_data, IP_size)
% create IP packet

FFFF = uint16(hex2dec('FFFF'));

version_IHL = uint8(69); % IPv4 and IP header length of 5
ToS = uint8(0); % no QOS on network

length = IP_size + uint16(20); % hardcode header length to 5

length_BE = (typecast(length, 'uint8')); % change to big endian
length_BE = length_BE(end:-1:1);

% counter
persistent ID % identification
if isempty(ID)
    ID = uint16(0);
else
    ID = ID + 1;
end

ff = [ uint8(bin2dec('01000000')) 0 ]; % don't fragment packets

TTL = uint8(10); % ttl to 10 seconds/hops

protocol = uint8(hex2dec('11')); % UDP Protocol


header = [ version_IHL ToS length_BE typecast(ID, 'uint8') ff TTL protocol 0 0 sourceIP destIP];

% header(11:12) = typecast(bitcmp(uint16(sum( typecast(bitcmp(header), 'uint16') ))), 'uint8'); % checksum

checksum = FFFF - uint16(mod( uint32(sum( typecast(header, 'uint16') )), uint32(FFFF) ));
header(11:12) = typecast(checksum, 'uint8');

packet = [ header IP_data ];

== matlab function rigPeripheralNet/Screen/Screen - Data/MATLAB Function ==
  data: u input; y output
function y = padData(u)

z = uint8(zeros(1434, 1))';

z(1:length(u)) = u;

y = z';

== matlab function rigPeripheralNet/Screen/Screen - Data/Make UDP Packet/Add IP Header ==
  data: sourceIP input uint8 size=[1 4]; packet output uint8; destIP input uint8 size=[1 4]; IP_data input uint8; IP_size input uint16 size=[1 1]; length output uint16 size=[1 1]
function [packet, length] = makeIP(sourceIP, destIP, IP_data, IP_size)
% create IP packet

FFFF = uint16(hex2dec('FFFF'));

version_IHL = uint8(69); % IPv4 and IP header length of 5
ToS = uint8(0); % no QOS on network

length = IP_size + uint16(20); % hardcode header length to 5

length_BE = (typecast(length, 'uint8')); % change to big endian
length_BE = length_BE(end:-1:1);

% counter
persistent ID % identification
if isempty(ID)
    ID = uint16(0);
else
    ID = ID + 1;
end

ff = [ uint8(bin2dec('01000000')) 0 ]; % don't fragment packets

TTL = uint8(10); % ttl to 10 seconds/hops

protocol = uint8(hex2dec('11')); % UDP Protocol


header = [ version_IHL ToS length_BE typecast(ID, 'uint8') ff TTL protocol 0 0 sourceIP destIP];

% header(11:12) = typecast(bitcmp(uint16(sum( typecast(bitcmp(header), 'uint16') ))), 'uint8'); % checksum

checksum = FFFF - uint16(mod( uint32(sum( typecast(header, 'uint16') )), uint32(FFFF) ));
header(11:12) = typecast(checksum, 'uint8');

packet = [ header IP_data ];

== matlab function rigPeripheralNet/Screen/Screen - Data/Make UDP Packet/Add UDP Header ==
  data: sourceIP input uint8 size=[1 4]; packet output; destIP input uint8 size=[1 4]; sourcePort input uint16 size=[1 1]; destPort input uint16 size=[1 1]; UDP_data input uint8; UDP_size input uint16 size=[1 1]; length output uint16 size=[1 1]
function [packet, length] = makeUDP(sourceIP, destIP, sourcePort, destPort, UDP_data, UDP_size)
% create UDP packet

% sourceIP and destIP are 1x4 uint8 of the IP (in address order)
% sourcePort and destPort are uint16
% UDP_data is uint8 of 1xN packet data
% UDP_size is uint16 size of UDP_data
%
% NOTE: UDP_size MUST BE EVEN
FFFF = uint16(hex2dec('FFFF'));

protocol = uint8(hex2dec('11'));

length = UDP_size + uint16(8);

length_BE = (typecast(length, 'uint8')); % flip to big endian
length_BE = length_BE(end:-1:1);

sourcePort_BE = (typecast(sourcePort, 'uint8'));
sourcePort_BE = sourcePort_BE(end:-1:1);

destPort_BE   = (typecast(destPort,   'uint8'));
destPort_BE = destPort_BE(end:-1:1);

header = [sourcePort_BE destPort_BE length_BE uint8([0 0])];

pseudoHeader = [sourceIP destIP uint8(0) protocol length_BE];

% header(7:8) = typecast( bitcmp(uint16(sum( typecast(bitcmp([pseudoHeader header UDP_data]), 'uint16') ))), 'uint8');


checksum = FFFF - uint16(mod( uint32(sum( typecast([pseudoHeader header UDP_data], 'uint16') )), uint32(FFFF) ));
header(7:8) = typecast(checksum, 'uint8');

packet = [ header UDP_data ];

== matlab function rigPeripheralNet/Sound/Sound - Control/MATLAB Function ==
  data: u input; y output
function y = padData(u)

z = uint8(zeros(1434, 1))';

z(1:length(u)) = u;

y = z';

== matlab function rigPeripheralNet/Receive Most Recent Peripheral Packets/parsePackets/For Iterator Subsystem/Parse Cerebus UDP Packets ==
  data: laptopDataOut output Bus: peripheralData size=1; vizDataOut output Bus: peripheralData size=1; n input; data input uint8; length input; ipDest input; laptopIpSource input; laptopPortDest input; vizIpSource input; vizPortDest input; robotIpSource input; robotPortDest input; robotDataOut output Bus: peripheralData; windowsIpSource input; windowsPortDest input; windowsDataOut output Bus: peripheralData; windowsPC1IpSource input; windowsPC1PortDest input; windowsPC1DataOut output Bus: peripheralData; mouseDataOut output Bus: peripheralData; mouseDataIpSource input; mouseDataPortDest input
function [laptopDataOut, vizDataOut, robotDataOut, windowsDataOut, windowsPC1DataOut, mouseDataOut]  = ...
    parsePacketFromIP(n, data, length, ipDest, laptopIpSource, laptopPortDest, vizIpSource, vizPortDest, ...
        robotIpSource, robotPortDest, windowsIpSource, windowsPortDest, windowsPC1IpSource, windowsPC1PortDest, ...
            mouseDataIpSource, mouseDataPortDest)
%#codegen 

%%%%%%%%%%%%%%%%%%%%%%%%%%%%%
%
% parse for specific ip address
%
% Vikash 
% NPTL 
% Stanford University 
%
%%%%%%%%%%%%%%%%%%%%%%%%%%%%%

%%%%%%%%%%%%%%%%%%%%%%%%%%%%%
%
% Outputs:
%
% packetData - data from first packet to match this IP
% packetLength - length of the matching packet data
% 
%%%%%%%%%%%%%%%%%%%%%%%%%%%%%

persistent laptopData vizData robotData windowsData windowsPC1Data mouseData;

if(isempty(laptopData))
    laptopData.data = coder.nullcopy(uint8(zeros(1, 1400)));
    laptopData.dataLen = uint16(0);
    laptopData.receive = false;
    vizData.data = coder.nullcopy(uint8(zeros(1, 1400)));
    vizData.dataLen = uint16(0);
    vizData.receive = false;
    robotData.data = coder.nullcopy(uint8(zeros(1, 1400)));
    robotData.dataLen = uint16(0);
    robotData.receive = false;
    
    %from PC2, currently for smartnav Jan. 15 2018
    windowsData.data = coder.nullcopy(uint8(zeros(1, 1400)));
    windowsData.dataLen = uint16(0);
    windowsData.receive = false;
    
    %from PC1, tobii data + maybe smartnav if we want to switch Jan. 15
    %2018
    windowsPC1Data.data = coder.nullcopy(uint8(zeros(1, 1400)));
    windowsPC1Data.dataLen = uint16(0);
    windowsPC1Data.receive = false;
    
    %PC1 mouse input, for controlling the games with a mouse while also
    %tracking head/eye input from T5
    mouseData.data = coder.nullcopy(uint8(zeros(1, 1400)));
    mouseData.dataLen = uint16(0);
    mouseData.receive = false;
end

if(n == 1) % First loop for this tick, can't combine with persistent declarations
    laptopData.data = coder.nullcopy(uint8(zeros(1, 1400)));
    laptopData.dataLen = uint16(0);
    laptopData.receive = false;
    vizData.data = coder.nullcopy(uint8(zeros(1, 1400)));
    vizData.dataLen = uint16(0);
    vizData.receive = false;
    robotData.data = coder.nullcopy(uint8(zeros(1, 1400)));
    robotData.dataLen = uint16(0);
    robotData.receive = false;
    windowsData.data = coder.nullcopy(uint8(zeros(1, 1400)));
    windowsData.dataLen = uint16(0);
    windowsData.receive = false;
    windowsPC1Data.data = coder.nullcopy(uint8(zeros(1, 1400)));
    windowsPC1Data.dataLen = uint16(0);
    windowsPC1Data.receive = false;
    mouseData.data = coder.nullcopy(uint8(zeros(1, 1400)));
    mouseData.dataLen = uint16(0);
    mouseData.receive = false;
end

if(all(data(13:16) == laptopIpSource) ...
        && all(data(17:20) == ipDest) ...
        && all(laptopPortDest == typecast(data(24:-1:23), 'uint16')))
    laptopData.receive = true;
    laptopData.data = uint8(data');
    laptopData.dataLen = uint16(length);
end

if(all(data(13:16) == vizIpSource) ...
        && all(data(17:20) == ipDest) ...
        && all(vizPortDest == typecast(data(24:-1:23), 'uint16')))
    vizData.receive = true;
    vizData.data = uint8(data');
    vizData.dataLen = uint16(length);
end

if(all(data(13:16) == robotIpSource) ...
        && all(data(17:20) == ipDest) ...
        && all(robotPortDest == typecast(data(24:-1:23), 'uint16')))
    robotData.receive = true;
    robotData.data = uint8(data');
    robotData.dataLen = uint16(length);
end

if(all(data(13:16) == windowsIpSource) ...
        && all(data(17:20) == ipDest) ...
        && all(windowsPortDest == typecast(data(24:-1:23), 'uint16')))
    windowsData.receive = true;
    windowsData.data = uint8(data');
    windowsData.dataLen = uint16(length);
end

if(all(data(13:16) == windowsPC1IpSource) ...
        && all(data(17:20) == ipDest) ...
        && all(windowsPC1PortDest == typecast(data(24:-1:23), 'uint16')))
    windowsPC1Data.receive = true;
    windowsPC1Data.data = uint8(data');
    windowsPC1Data.dataLen = uint16(length);
end

if(all(data(13:16) == mouseDataIpSource) ...
        && all(data(17:20) == ipDest) ...
        && all(mouseDataPortDest == typecast(data(24:-1:23), 'uint16')))
    mouseData.receive = true;
    mouseData.data = uint8(data');
    mouseData.dataLen = uint16(length);
end

laptopDataOut = laptopData;
vizDataOut = vizData;
robotDataOut = robotData;
windowsDataOut = windowsData;
windowsPC1DataOut = windowsPC1Data;
mouseDataOut = mouseData;

== matlab function rigPeripheralNet/Sound/Sound - Control/Make UDP Packet/Add IP Header ==
  data: sourceIP input uint8 size=[1 4]; packet output uint8; destIP input uint8 size=[1 4]; IP_data input uint8; IP_size input uint16 size=[1 1]; length output uint16 size=[1 1]
function [packet, length] = makeIP(sourceIP, destIP, IP_data, IP_size)
% create IP packet

FFFF = uint16(hex2dec('FFFF'));

version_IHL = uint8(69); % IPv4 and IP header length of 5
ToS = uint8(0); % no QOS on network

length = IP_size + uint16(20); % hardcode header length to 5

length_BE = (typecast(length, 'uint8')); % change to big endian
length_BE = length_BE(end:-1:1);

% counter
persistent ID % identification
if isempty(ID)
    ID = uint16(0);
else
    ID = ID + 1;
end

ff = [ uint8(bin2dec('01000000')) 0 ]; % don't fragment packets

TTL = uint8(10); % ttl to 10 seconds/hops

protocol = uint8(hex2dec('11')); % UDP Protocol


header = [ version_IHL ToS length_BE typecast(ID, 'uint8') ff TTL protocol 0 0 sourceIP destIP];

% header(11:12) = typecast(bitcmp(uint16(sum( typecast(bitcmp(header), 'uint16') ))), 'uint8'); % checksum

checksum = FFFF - uint16(mod( uint32(sum( typecast(header, 'uint16') )), uint32(FFFF) ));
header(11:12) = typecast(checksum, 'uint8');

packet = [ header IP_data ];

== matlab function rigPeripheralNet/Screen/Screen - Control/Make UDP Packet/Add UDP Header ==
  data: sourceIP input uint8 size=[1 4]; packet output; destIP input uint8 size=[1 4]; sourcePort input uint16 size=[1 1]; destPort input uint16 size=[1 1]; UDP_data input uint8; UDP_size input uint16 size=[1 1]; length output uint16 size=[1 1]
function [packet, length] = makeUDP(sourceIP, destIP, sourcePort, destPort, UDP_data, UDP_size)
% create UDP packet

% sourceIP and destIP are 1x4 uint8 of the IP (in address order)
% sourcePort and destPort are uint16
% UDP_data is uint8 of 1xN packet data
% UDP_size is uint16 size of UDP_data
%
% NOTE: UDP_size MUST BE EVEN
FFFF = uint16(hex2dec('FFFF'));

protocol = uint8(hex2dec('11'));

length = UDP_size + uint16(8);

length_BE = (typecast(length, 'uint8')); % flip to big endian
length_BE = length_BE(end:-1:1);

sourcePort_BE = (typecast(sourcePort, 'uint8'));
sourcePort_BE = sourcePort_BE(end:-1:1);

destPort_BE   = (typecast(destPort,   'uint8'));
destPort_BE = destPort_BE(end:-1:1);

header = [sourcePort_BE destPort_BE length_BE uint8([0 0])];

pseudoHeader = [sourceIP destIP uint8(0) protocol length_BE];

% header(7:8) = typecast( bitcmp(uint16(sum( typecast(bitcmp([pseudoHeader header UDP_data]), 'uint16') ))), 'uint8');


checksum = FFFF - uint16(mod( uint32(sum( typecast([pseudoHeader header UDP_data], 'uint16') )), uint32(FFFF) ));
header(7:8) = typecast(checksum, 'uint8');

packet = [ header UDP_data ];

== matlab function rigPeripheralNet/request data from laptop/Laptop Data Request ==
  data: clock input uint32 size=1; send output; data output; dataLen output
function [send, data, dataLen] = laptopDataRequest(clock)
%#codegen

data = uint8(zeros(1, 500));
data(1:4) = typecast(clock, 'uint8');
dataLen = uint16(length(data));

% Transmit 12 serial bytes every 100 ms
if(mod(clock, 10)==0)
    send = true;
else
    send = false;
end

send = true;

== matlab function rigPeripheralNet/Sound/Sound - Control/Make UDP Packet/Add UDP Header ==
  data: sourceIP input uint8 size=[1 4]; packet output; destIP input uint8 size=[1 4]; sourcePort input uint16 size=[1 1]; destPort input uint16 size=[1 1]; UDP_data input uint8; UDP_size input uint16 size=[1 1]; length output uint16 size=[1 1]
function [packet, length] = makeUDP(sourceIP, destIP, sourcePort, destPort, UDP_data, UDP_size)
% create UDP packet

% sourceIP and destIP are 1x4 uint8 of the IP (in address order)
% sourcePort and destPort are uint16
% UDP_data is uint8 of 1xN packet data
% UDP_size is uint16 size of UDP_data
%
% NOTE: UDP_size MUST BE EVEN
FFFF = uint16(hex2dec('FFFF'));

protocol = uint8(hex2dec('11'));

length = UDP_size + uint16(8);

length_BE = (typecast(length, 'uint8')); % flip to big endian
length_BE = length_BE(end:-1:1);

sourcePort_BE = (typecast(sourcePort, 'uint8'));
sourcePort_BE = sourcePort_BE(end:-1:1);

destPort_BE   = (typecast(destPort,   'uint8'));
destPort_BE = destPort_BE(end:-1:1);

header = [sourcePort_BE destPort_BE length_BE uint8([0 0])];

pseudoHeader = [sourceIP destIP uint8(0) protocol length_BE];

% header(7:8) = typecast( bitcmp(uint16(sum( typecast(bitcmp([pseudoHeader header UDP_data]), 'uint16') ))), 'uint8');


checksum = FFFF - uint16(mod( uint32(sum( typecast([pseudoHeader header UDP_data], 'uint16') )), uint32(FFFF) ));
header(7:8) = typecast(checksum, 'uint8');

packet = [ header UDP_data ];

== matlab function rigPeripheralNet/Sound/Sound - Data/MATLAB Function ==
  data: u input; y output
function y = padData(u)

z = uint8(zeros(1434, 1))';

z(1:length(u)) = u;

y = z';

== matlab function rigPeripheralNet/Sound/Sound - Data/Make UDP Packet/Add IP Header ==
  data: sourceIP input uint8 size=[1 4]; packet output uint8; destIP input uint8 size=[1 4]; IP_data input uint8; IP_size input uint16 size=[1 1]; length output uint16 size=[1 1]
function [packet, length] = makeIP(sourceIP, destIP, IP_data, IP_size)
% create IP packet

FFFF = uint16(hex2dec('FFFF'));

version_IHL = uint8(69); % IPv4 and IP header length of 5
ToS = uint8(0); % no QOS on network

length = IP_size + uint16(20); % hardcode header length to 5

length_BE = (typecast(length, 'uint8')); % change to big endian
length_BE = length_BE(end:-1:1);

% counter
persistent ID % identification
if isempty(ID)
    ID = uint16(0);
else
    ID = ID + 1;
end

ff = [ uint8(bin2dec('01000000')) 0 ]; % don't fragment packets

TTL = uint8(10); % ttl to 10 seconds/hops

protocol = uint8(hex2dec('11')); % UDP Protocol


header = [ version_IHL ToS length_BE typecast(ID, 'uint8') ff TTL protocol 0 0 sourceIP destIP];

% header(11:12) = typecast(bitcmp(uint16(sum( typecast(bitcmp(header), 'uint16') ))), 'uint8'); % checksum

checksum = FFFF - uint16(mod( uint32(sum( typecast(header, 'uint16') )), uint32(FFFF) ));
header(11:12) = typecast(checksum, 'uint8');

packet = [ header IP_data ];

== matlab function rigPeripheralNet/Sound/Sound - Data/Make UDP Packet/Add UDP Header ==
  data: sourceIP input uint8 size=[1 4]; packet output; destIP input uint8 size=[1 4]; sourcePort input uint16 size=[1 1]; destPort input uint16 size=[1 1]; UDP_data input uint8; UDP_size input uint16 size=[1 1]; length output uint16 size=[1 1]
function [packet, length] = makeUDP(sourceIP, destIP, sourcePort, destPort, UDP_data, UDP_size)
% create UDP packet

% sourceIP and destIP are 1x4 uint8 of the IP (in address order)
% sourcePort and destPort are uint16
% UDP_data is uint8 of 1xN packet data
% UDP_size is uint16 size of UDP_data
%
% NOTE: UDP_size MUST BE EVEN
FFFF = uint16(hex2dec('FFFF'));

protocol = uint8(hex2dec('11'));

length = UDP_size + uint16(8);

length_BE = (typecast(length, 'uint8')); % flip to big endian
length_BE = length_BE(end:-1:1);

sourcePort_BE = (typecast(sourcePort, 'uint8'));
sourcePort_BE = sourcePort_BE(end:-1:1);

destPort_BE   = (typecast(destPort,   'uint8'));
destPort_BE = destPort_BE(end:-1:1);

header = [sourcePort_BE destPort_BE length_BE uint8([0 0])];

pseudoHeader = [sourceIP destIP uint8(0) protocol length_BE];

% header(7:8) = typecast( bitcmp(uint16(sum( typecast(bitcmp([pseudoHeader header UDP_data]), 'uint16') ))), 'uint8');


checksum = FFFF - uint16(mod( uint32(sum( typecast([pseudoHeader header UDP_data], 'uint16') )), uint32(FFFF) ));
header(7:8) = typecast(checksum, 'uint8');

packet = [ header UDP_data ];

== matlab function rigPeripheralNet/Asynch/Asynch - Control/MATLAB Function ==
  data: u input; y output
function y = padData(u)

z = uint8(zeros(1434, 1))';

z(1:length(u)) = u;

y = z';

== matlab function rigPeripheralNet/Asynch/Asynch - Control/Make UDP Packet/Add IP Header ==
  data: sourceIP input uint8 size=[1 4]; packet output uint8; destIP input uint8 size=[1 4]; IP_data input uint8; IP_size input uint16 size=[1 1]; length output uint16 size=[1 1]
function [packet, length] = makeIP(sourceIP, destIP, IP_data, IP_size)
% create IP packet

FFFF = uint16(hex2dec('FFFF'));

version_IHL = uint8(69); % IPv4 and IP header length of 5
ToS = uint8(0); % no QOS on network

length = IP_size + uint16(20); % hardcode header length to 5

length_BE = (typecast(length, 'uint8')); % change to big endian
length_BE = length_BE(end:-1:1);

% counter
persistent ID % identification
if isempty(ID)
    ID = uint16(0);
else
    ID = ID + 1;
end

ff = [ uint8(bin2dec('01000000')) 0 ]; % don't fragment packets

TTL = uint8(10); % ttl to 10 seconds/hops

protocol = uint8(hex2dec('11')); % UDP Protocol


header = [ version_IHL ToS length_BE typecast(ID, 'uint8') ff TTL protocol 0 0 sourceIP destIP];

% header(11:12) = typecast(bitcmp(uint16(sum( typecast(bitcmp(header), 'uint16') ))), 'uint8'); % checksum

checksum = FFFF - uint16(mod( uint32(sum( typecast(header, 'uint16') )), uint32(FFFF) ));
header(11:12) = typecast(checksum, 'uint8');

packet = [ header IP_data ];
